simulink model "discrete"  (R2017a)
settings: Solver=VariableStepAuto  StartTime=0.0  StopTime=20.0  RelTol=1e-3
undefined symbols (not defined in the file or in its folder): DiscIntNeverNeededParam
settings Model: Creator=aous  LastModifiedBy=aous

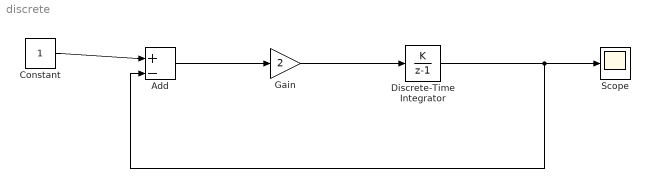
== system discrete ==
  Add : Sum  Inputs=+|-
  Constant : Constant
  Discrete-Time Integrator : DiscreteIntegrator  IntegratorMethod=Accumulation: Forward Euler  gainval=0.1  InitialConditionSetting=State (most efficient)  SampleTime=0.1  ICPrevOutput=DiscIntNeverNeededParam  ICPrevScaledInput=DiscIntNeverNeededParam
  Gain : Gain  Gain=2
  Scope : Scope
  wires:
  Gain/1 -> Discrete-Time Integrator/1
  Constant/1 -> Add/1
  Add/1 -> Gain/1
  Discrete-Time Integrator/1 -> Scope/1, Add/2
